simulink model "rcrc_sim"  (R2024a)
settings: Solver=ode23tb  StartTime=0.0  StopTime=0.1  RelTol=1e-3
values from neighbouring files (symbols this model uses):
  A = [-((R1+R2)/(R1*R2*C1)), 1/(R2*C1); 1/(R2*C2), -1/(R2*C2)]    [rcrc_ini.m]
  B = [1/(R1*C1); 0]    [rcrc_ini.m]
  C = [0, 1]    [rcrc_ini.m]
  C1 = 470e-9    (= 4.7e-07)    [rcrc_ini.m]
  C2 = C1    (= 4.7e-07)    [rcrc_ini.m]
  H = place(A', C', 3*ew)'    [rcrc_ini.m]
  K = place(A, B, ew)    [rcrc_ini.m]
  R1 = 4.7e3    (= 4700)    [rcrc_ini.m]
  R2 = R1    (= 4700)    [rcrc_ini.m]
  V = 1/dcgain(sys_cl)    [rcrc_ini.m]
settings Model: Creator=pmic  LastModifiedBy=nikla
settings SolverCC: AlgebraicLoopSolver=TrustRegion
settings DebuggingCC: UnconnectedInputMsg=warning  UnconnectedOutputMsg=warning  UnconnectedLineMsg=warning
settings ModelReferenceCC: EnableRefExpFcnMdlSchedulingChecks=on
settings RTWCC: GPUComputeCapability=3.5  DLArmComputeVersion=19.05

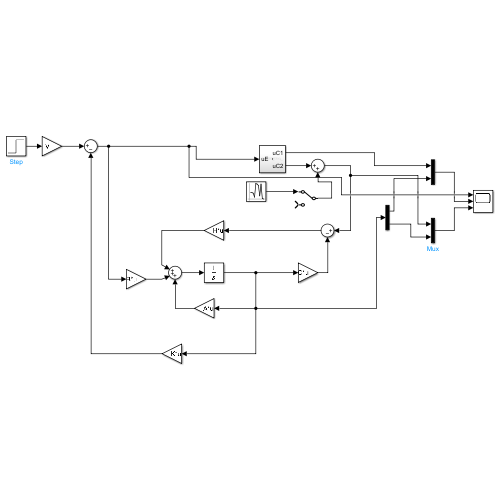
[thumbnail: Simulink's stored preview of the top-level diagram]
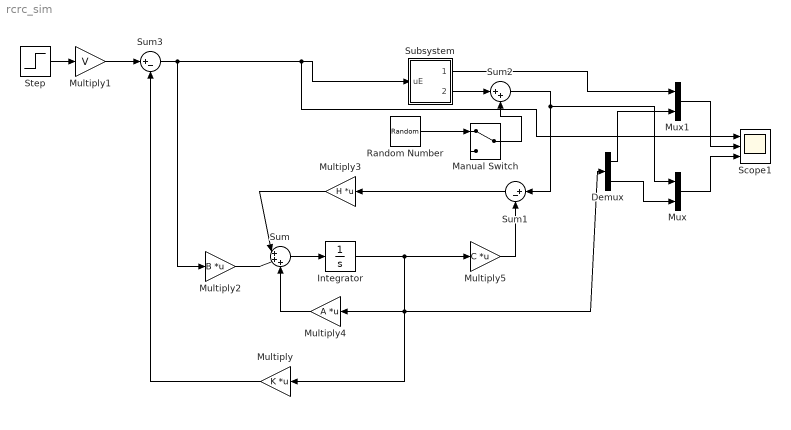
== system rcrc_sim ==
  Demux : Demux  Outputs=2
  Integrator : Integrator
  Manual Switch : ManualSwitch
  Multiply : Gain  Gain=K  Multiplication=Matrix(K*u)
  Multiply1 : Gain  Gain=V
  Multiply2 : Gain  Gain=B  Multiplication=Matrix(K*u)
  Multiply3 : Gain  Gain=H  Multiplication=Matrix(K*u)
  Multiply4 : Gain  Gain=A  Multiplication=Matrix(K*u)
  Multiply5 : Gain  Gain=C  Multiplication=Matrix(K*u)
  Mux : Mux  Inputs=2
  Mux1 : Mux  Inputs=2
  Random Number : RandomNumber  Variance=0.001  SampleTime=0.0001
  Scope1 : Scope  NumInputPorts=3
  Step : Step  Time=0.01  SampleTime=0
  Subsystem : Subsystem
  Sum : Sum  Inputs=|+++
  Sum1 : Sum  Inputs=|+-
  Sum2 : Sum  Inputs=|++
  Sum3 : Sum  Inputs=|+-
  wires:
  Subsystem/1(uC1) -> Mux1/1
  Sum3/1 -> Scope1/1, Subsystem/1(uE), Multiply2/1
  Multiply/1 -> Sum3/2
  Step/1 -> Multiply1/1
  Sum2/1 -> Mux/1, Sum1/1
  Multiply1/1 -> Sum3/1
  Sum/1 -> Integrator/1
  Multiply2/1 -> Sum/2
  Multiply3/1 -> Sum/1
  Multiply4/1 -> Sum/3
  Integrator/1 -> Multiply4/1, Multiply/1, Demux/1, Multiply5/1
  Sum1/1 -> Multiply3/1
  Multiply5/1 -> Sum1/2
  Random Number/1 -> Manual Switch/1
  Subsystem/2(uC2) -> Sum2/1
  Manual Switch/1 -> Sum2/2
  Demux/1 -> Mux1/2
  Demux/2 -> Mux/2
  Mux1/1 -> Scope1/2
  Mux/1 -> Scope1/3

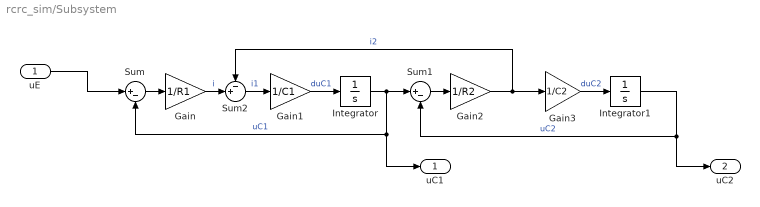
== system rcrc_sim/Subsystem ==
  uE : Inport
  Gain : Gain  Gain=1/R1
  Gain1 : Gain  Gain=1/C1
  Gain2 : Gain  Gain=1/R2
  Gain3 : Gain  Gain=1/C2
  Integrator : Integrator
  Integrator1 : Integrator
  Sum : Sum  Inputs=|+-
  Sum1 : Sum  Inputs=|+-
  Sum2 : Sum  Inputs=-+|
  uC1 : Outport
  uC2 : Outport  Port=2
  wires:
  Sum/1 -> Gain/1
  Gain1/1 -> Integrator/1  "duC1"
  uE/1 -> Sum/1
  Gain/1 -> Sum2/2  "i"
  Sum2/1 -> Gain1/1  "i1"
  Gain3/1 -> Integrator1/1  "duC2"
  Integrator1/1 -> uC2/1, Sum1/2  "uC2"
  Integrator/1 -> uC1/1, Sum/2, Sum1/1  "uC1"
  Sum1/1 -> Gain2/1
  Gain2/1 -> Gain3/1, Sum2/1  "i2"
